simulink library "ESTS_WHL"  (R2024b)
settings: Solver=VariableStepAuto  StartTime=0.0  StopTime=10.0  RelTol=1e-3
settings Model: Creator=blatak  LastModifiedBy=blatak

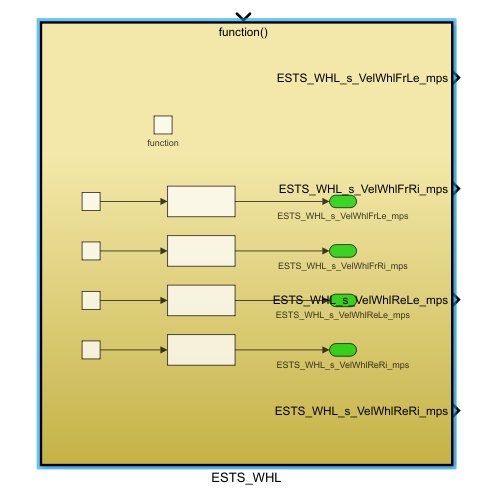
[thumbnail: Simulink's stored preview of the top-level diagram]
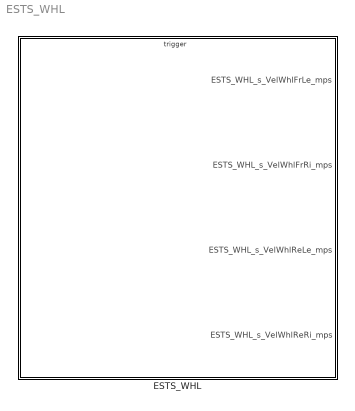
== system ESTS_WHL ==
  ESTS_WHL : Subsystem  TreatAsAtomicUnit=on

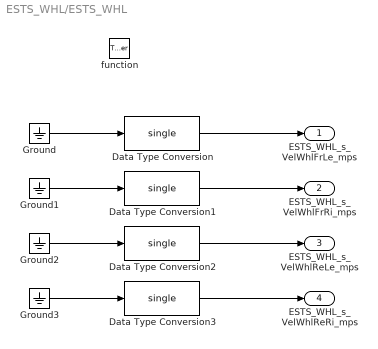
== system ESTS_WHL/ESTS_WHL ==
  function : TriggerPort  TriggerType=function-call  VariantControl=(inherit)
  Data Type Conversion{,1..3} (4 alike) : DataTypeConversion  OutDataTypeStr=single  SaturateOnIntegerOverflow=off  RndMeth=Floor
  Ground{,1..3} (4 alike) : Ground
  ESTS_WHL_s_VelWhlFrLe_mps : Outport
  ESTS_WHL_s_VelWhlFrRi_mps : Outport  Port=2
  ESTS_WHL_s_VelWhlReLe_mps : Outport  Port=3
  ESTS_WHL_s_VelWhlReRi_mps : Outport  Port=4
  wires:
  Data Type Conversion/1 -> ESTS_WHL_s_VelWhlFrLe_mps/1
  Ground/1 -> Data Type Conversion/1
  Data Type Conversion1/1 -> ESTS_WHL_s_VelWhlFrRi_mps/1
  Ground1/1 -> Data Type Conversion1/1
  Data Type Conversion2/1 -> ESTS_WHL_s_VelWhlReLe_mps/1
  Ground2/1 -> Data Type Conversion2/1
  Data Type Conversion3/1 -> ESTS_WHL_s_VelWhlReRi_mps/1
  Ground3/1 -> Data Type Conversion3/1
